simulink model "tres_test_distributedfuncts_df"  (R2014a)
settings: Solver=VariableStepDiscrete  StartTime=0.0  StopTime=60  RelTol=1e-3
libraries: tres_simulink_blockset x10
settings Model: Creator=matteo  LastModifiedBy=MM244911
settings DataIOCC: SignalLoggingSaveFormat=ModelDataLogs
settings OptimizationCC: ExpressionDepthLimit=2147483647
settings DebuggingCC: UnderspecifiedInitializationDetection=Classic  FcnCallInpInsideContextMsg=EnableAllAsWarning  StateNameClashWarn=warning

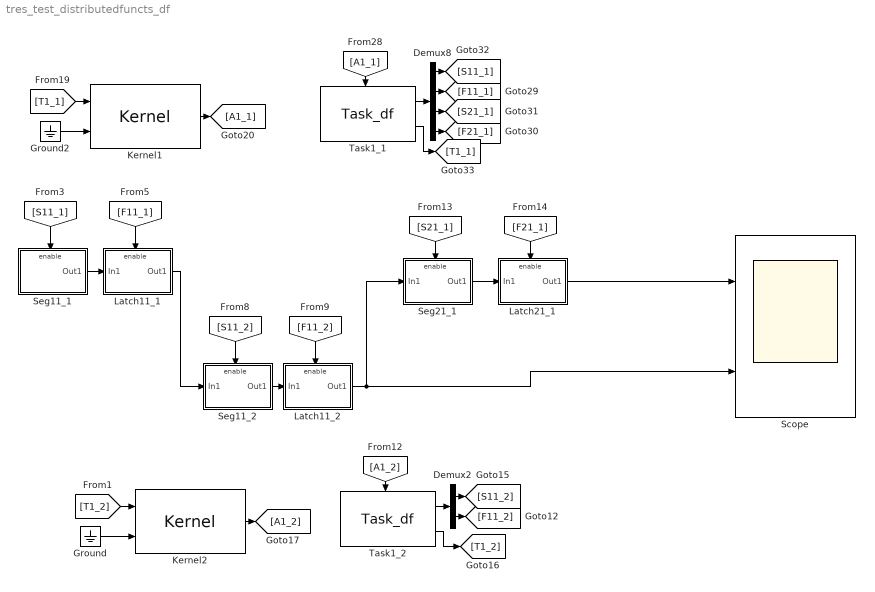
== system tres_test_distributedfuncts_df ==
  Demux2 : Demux  Outputs=2
  Demux8 : Demux
  Ground : Ground
  Ground2 : Ground
  Kernel1 : tres_simulink_blockset/Kernel  taskset_descr_name=task_set_descr1  scheduling_policy=DEADLINE_MONOTONIC  dead_miss_rule=Continue  time_res=Milli_Seconds  core_num=1  under_engine=RTSIM
  Kernel2 : tres_simulink_blockset/Kernel  taskset_descr_name=task_set_descr2  scheduling_policy=DEADLINE_MONOTONIC  dead_miss_rule=Continue  time_res=Milli_Seconds  core_num=1  under_engine=RTSIM
  Latch11_1 : Subsystem
  Latch11_2 : Subsystem
  Latch21_1 : Subsystem
  Scope : Scope  NumInputPorts=2
      settings: YMin=-5~-5  YMax=5~5
  Seg11_1 : Subsystem  TreatAsAtomicUnit=on
  Seg11_2 : Subsystem
  Seg21_1 : Subsystem
  Task1_1 : tres_simulink_blockset/Task_df  conf_name=t11_instrs
  Task1_2 : tres_simulink_blockset/Task_df  conf_name=t12_instrs
  wires:
  Ground/1 -> Kernel2/2
  Kernel2/1 -> [A1_2]
  Task1_2/2 -> [T1_2]
  Demux2/1 -> [S11_2]
  Demux2/2 -> [F11_2]
  Task1_2/1 -> Demux2/1
  [A1_2] -> Task1_2/Trigger
  [F21_1] -> Latch21_1/Enable
  [S21_1] -> Seg21_1/Enable
  [T1_1] -> Kernel1/1
  Ground2/1 -> Kernel1/2
  Kernel1/1 -> [A1_1]
  Task1_1/2 -> [T1_1]
  Task1_1/1 -> Demux8/1
  Demux8/1 -> [S11_1]
  Demux8/2 -> [F11_1]
  Demux8/4 -> [F21_1]
  Demux8/3 -> [S21_1]
  [T1_2] -> Kernel2/1
  Latch21_1/1(Out1) -> Scope/1
  [S11_1] -> Seg11_1/Enable
  Seg11_1/1(Out1) -> Latch11_1/1(In1)
  Latch11_1/1(Out1) -> Seg11_2/1(In1)
  [S11_2] -> Seg11_2/Enable
  Latch11_2/1(Out1) -> Seg21_1/1(In1), Scope/2
  [F11_2] -> Latch11_2/Enable
  Seg11_2/1(Out1) -> Latch11_2/1(In1)
  Seg21_1/1(Out1) -> Latch21_1/1(In1)
  [F11_1] -> Latch11_1/Enable
  [A1_1] -> Task1_1/Trigger

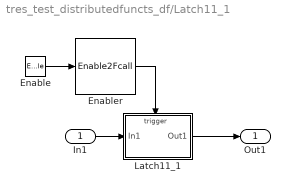
== system tres_test_distributedfuncts_df/Latch11_1 ==
  In1 : Inport
  Enable : EnablePort  ShowOutputPort=on
  Enabler : tres_simulink_blockset/Enable2Fcall
  Latch11_1 : Subsystem  TreatAsAtomicUnit=on
  Out1 : Outport
  wires:
  In1/1 -> Latch11_1/1(In1)
  Latch11_1/1(Out1) -> Out1/1
  Enable/1 -> Enabler/1
  Enabler/1 -> Latch11_1/Trigger

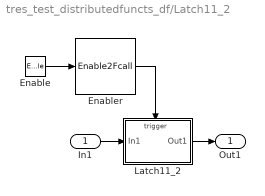
== system tres_test_distributedfuncts_df/Latch11_2 ==
  In1 : Inport
  Enable : EnablePort  ShowOutputPort=on
  Enabler : tres_simulink_blockset/Enable2Fcall
  Latch11_2 : Subsystem  TreatAsAtomicUnit=on
  Out1 : Outport
  wires:
  In1/1 -> Latch11_2/1(In1)
  Latch11_2/1(Out1) -> Out1/1
  Enable/1 -> Enabler/1
  Enabler/1 -> Latch11_2/Trigger

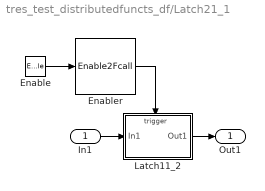
== system tres_test_distributedfuncts_df/Latch21_1 ==
  In1 : Inport
  Enable : EnablePort  ShowOutputPort=on
  Enabler : tres_simulink_blockset/Enable2Fcall
  Latch11_2 : Subsystem  TreatAsAtomicUnit=on
  Out1 : Outport
  wires:
  In1/1 -> Latch11_2/1(In1)
  Latch11_2/1(Out1) -> Out1/1
  Enable/1 -> Enabler/1
  Enabler/1 -> Latch11_2/Trigger

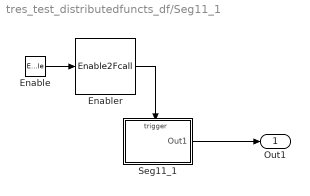
== system tres_test_distributedfuncts_df/Seg11_1 ==
  Enable : EnablePort  ShowOutputPort=on
  Enabler : tres_simulink_blockset/Enable2Fcall
  Seg11_1 : Subsystem  TreatAsAtomicUnit=on
  Out1 : Outport
  wires:
  Seg11_1/1(Out1) -> Out1/1
  Enable/1 -> Enabler/1
  Enabler/1 -> Seg11_1/Trigger

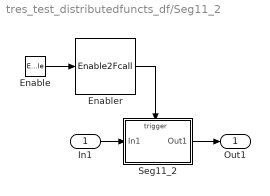
== system tres_test_distributedfuncts_df/Seg11_2 ==
  In1 : Inport
  Enable : EnablePort  ShowOutputPort=on
  Enabler : tres_simulink_blockset/Enable2Fcall
  Seg11_2 : Subsystem  TreatAsAtomicUnit=on
  Out1 : Outport
  wires:
  Seg11_2/1(Out1) -> Out1/1
  In1/1 -> Seg11_2/1(In1)
  Enable/1 -> Enabler/1
  Enabler/1 -> Seg11_2/Trigger

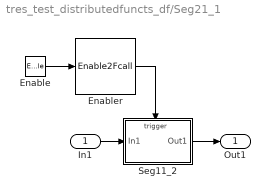
== system tres_test_distributedfuncts_df/Seg21_1 ==
  In1 : Inport
  Enable : EnablePort  ShowOutputPort=on
  Enabler : tres_simulink_blockset/Enable2Fcall
  Seg11_2 : Subsystem  TreatAsAtomicUnit=on
  Out1 : Outport
  wires:
  Seg11_2/1(Out1) -> Out1/1
  In1/1 -> Seg11_2/1(In1)
  Enable/1 -> Enabler/1
  Enabler/1 -> Seg11_2/Trigger

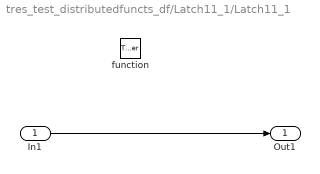
== system tres_test_distributedfuncts_df/Latch11_1/Latch11_1 ==
  In1 : Inport
  function : TriggerPort  TriggerType=function-call
  Out1 : Outport
  wires:
  In1/1 -> Out1/1

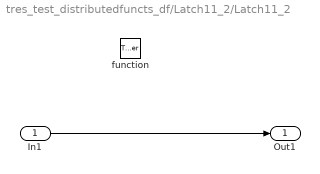
== system tres_test_distributedfuncts_df/Latch11_2/Latch11_2 ==
  In1 : Inport
  function : TriggerPort  TriggerType=function-call
  Out1 : Outport
  wires:
  In1/1 -> Out1/1

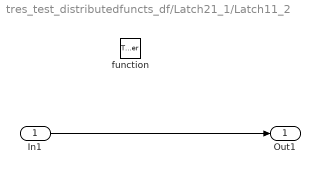
== system tres_test_distributedfuncts_df/Latch21_1/Latch11_2 ==
  In1 : Inport
  function : TriggerPort  TriggerType=function-call
  Out1 : Outport
  wires:
  In1/1 -> Out1/1

== system tres_test_distributedfuncts_df/Seg11_1/Seg11_1 ==
  function : TriggerPort  TriggerType=function-call
  Digital Clock : DigitalClock  SampleTime=-1
  Out1 : Outport
  wires:
  Digital Clock/1 -> Out1/1

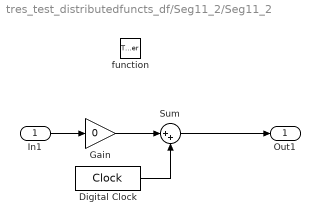
== system tres_test_distributedfuncts_df/Seg11_2/Seg11_2 ==
  In1 : Inport
  function : TriggerPort  TriggerType=function-call
  Digital Clock : DigitalClock  SampleTime=-1
  Gain : Gain  Gain=0
  Sum : Sum  Inputs=|++
  Out1 : Outport
  wires:
  Sum/1 -> Out1/1
  Digital Clock/1 -> Sum/2
  In1/1 -> Gain/1
  Gain/1 -> Sum/1

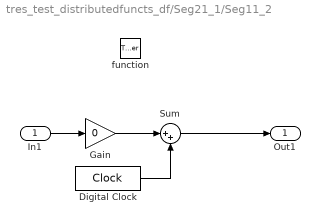
== system tres_test_distributedfuncts_df/Seg21_1/Seg11_2 ==
  In1 : Inport
  function : TriggerPort  TriggerType=function-call
  Digital Clock : DigitalClock  SampleTime=-1
  Gain : Gain  Gain=0
  Sum : Sum  Inputs=|++
  Out1 : Outport
  wires:
  Sum/1 -> Out1/1
  Digital Clock/1 -> Sum/2
  In1/1 -> Gain/1
  Gain/1 -> Sum/1
